simulink model "PV_SEPIC"  (R2025a)
settings: Solver=FixedStepAuto  StartTime=0.0  StopTime=3  RelTol=1e-3
undefined symbols (not defined in the file): Down, sigbuilder_block, Up
libraries: spsSeriesRLCBranchLib x6, spsVoltageMeasurementLib x3, spsGroundLib x2, eePwmGenerator x2, spsCurrentMeasurementLib x1, spsDiodeLib x1, spsMosfetLib x1, slpidlib x1, spsPVArrayLib x1, simulink x1, sps_lib x1
settings Model: Creator=gamezebra  LastModifiedBy=gamezebra

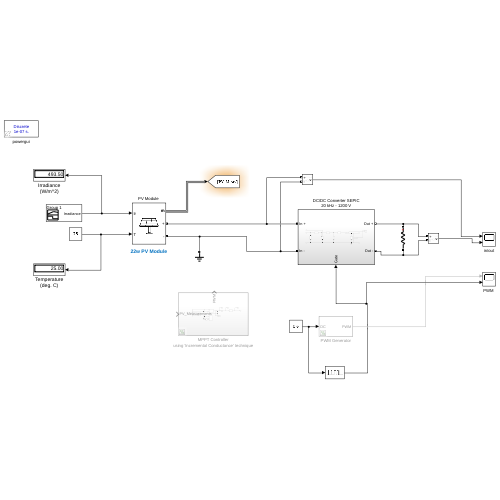
[thumbnail: Simulink's stored preview of the top-level diagram]
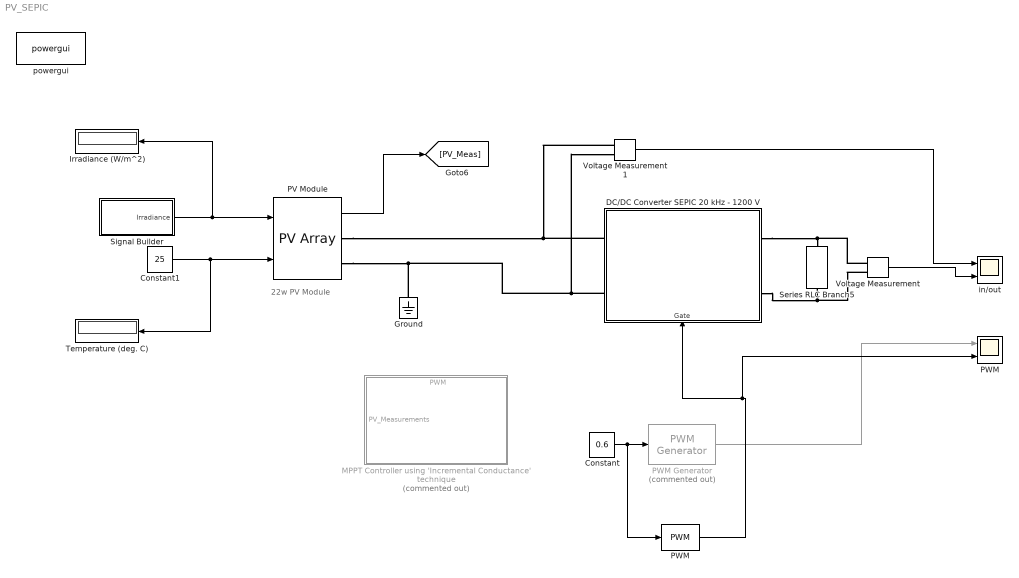
== system PV_SEPIC ==
  note: 22w PV Module
  Constant : Constant  Value=0.6
  Constant1 : Constant  Value=25
  DC/DC Converter SEPIC 20 kHz - 1200 V : Subsystem
      settings: PortSchema="{\"entries\":[{\"content\":{\"sides\":[{\"content\":{\"connectorIds\":[\"LConn1\",\"LConn2\"]},\"type\":\"ConnectorPlacement.EquallySpacedRectSide\",\"uuid\":\"91feb529-5820-4edf-8d0e-1c637fed9421\"},{\"content\":{\"connectorIds\":[\"RConn1\",\"RConn2\"],\"side\":\"RIGHT\"},\"type\":\"ConnectorPlacement.EquallySpacedRectSide\",\"uuid\":\"b4099113-c0ef-4c50-8083-88b14b98cc04\"},{\"content\":{\"side\":\"TOP\"},\"type\":\"ConnectorPlacement.EquallySpacedRectSide\",\"uuid\":\"250c6351-2de3-43d7-b6c9-3c3ed0452184\"},{\"content\":{\"connectorIds\":[\"In1\"],\"side\":\"BOTTOM\"},\"type\":\"ConnectorPlacement.EquallySpacedRectSide\",\"uuid\":\"484af620-bbf2-4328-991e-a08b15b59058\"}]},\"type\":\"ConnectorPlacement.EquallySpacedConnector\",\"uuid\":\"7041a545-1967-46d5-8643-e26f6c990daf\"}],\"packageUris\":[\"http://schema.mathworks.com/mf0/Connector/R2020b\"],\"version\":\"1.0\"}"
  Ground : spsGroundLib/Ground  LConnTagsString=a
  Irradiance (W/m^2) : Display
      settings: Format=bank  Decimation=1000
  MPPT Controller using 'Incremental Conductance' technique : Subsystem  Commented=on
      settings: PortSchema="{\"entries\":[{\"content\":{\"sides\":[{\"content\":{\"connectorIds\":[\"In1\"]},\"type\":\"ConnectorPlacement.EquallySpacedRectSide\",\"uuid\":\"beb56f4d-244a-4861-aa2c-056548243ef9\"},{\"content\":{\"side\":\"RIGHT\"},\"type\":\"ConnectorPlacement.EquallySpacedRectSide\",\"uuid\":\"efb26265-76c3-4ef7-8964-6d49d0ce5848\"},{\"content\":{\"connectorIds\":[\"Out1\"],\"side\":\"TOP\"},\"type\":\"ConnectorPlacement.EquallySpacedRectSide\",\"uuid\":\"f52004c3-ad48-43ff-bda9-03bf57742bdf\"}]},\"type\":\"ConnectorPlacement.EquallySpacedConnector\",\"uuid\":\"0b23e1d0-3529-41b8-bd5c-87ef798e8ebf\"}],\"packageUris\":[\"http://schema.mathworks.com/mf0/Connector/R2020b\"],\"version\":\"1.0\"}"
  "PV Module " : spsPVArrayLib/PV Array  Npar=1  Nser=1  PlotType=one module @ 25 deg.C & specified irradiances  S_vec="[ 1000  500  200 ]"  Temp_C_vec=25  ModuleName=User-defined  PlotWhenSelected=off  Pm=21.6138  Ncell=30  Voc=17.76  Isc=1.5  Vm=16.3  Im=1.326  beta_Voc_pc=-0.37  alpha_Isc_pc=0.07  beta_Voc=-0.065712  alpha_Isc=0.00105  IL=1.5  I0=2.021e-11  nI=1.0007  Rsh=187.3567  Rs=0.40236  RobustModel=off  RobustCellTemperature=313.3991  BAL=on  Tc=1e-6  Tfilter=5e-5
  PWM : simulink/Discontinuities/PWM  DisableCoverage=on  Period=1/100000  InitialDelay=0  DisallowZeroDutyCycle=off  RunAtFixedTimeIntervals=on  SampleTime=0.0000001
  "PWM " : Scope  NumInputPorts=2
      settings: Title=PWM  ActiveDisplayYMinimum=0.19673605992835486  ActiveDisplayYMaximum=1.3583645624515657  YLabel=Amplitudo
  PWM Generator : eePwmGenerator/PWM Generator  Commented=on  CarrCount=Up-Down  Tper=1/20000  Tdelay=0  Ts=0.001
  Series RLC Branch5 : spsSeriesRLCBranchLib/Series RLC Branch  LConnTagsString=__new0  RConnTagsString=__new0  BranchType=R  Resistance=25  Inductance=1e-3  SetiL0=off  InitialCurrent=0  Capacitance=5000e-6  Setx0=off  InitialVoltage=0  Measurements=None
  Signal Builder : Subsystem  Tag=STV Subsys  LoadFcn=sigbuilder_block('load');  StartFcn=sigbuilder_block('start');  StopFcn=sigbuilder_block('stop');  ClipboardFcn=sigbuilder_block('clipboard');  mask(Sigbuilder block){tuvar=[0:10]}
      mask help: Simulink:masks:SigbuilderBlock_MD
      mask init:
      | if ~strcmp(get_param(bdroot(gcbh),'SimulationStatus'),'stopped') tuvar = sigbuilder_block('maskInit'); end
      settings: CopyFcn=sigbuilder_block('copy');  DeleteFcn=sigbuilder_block('delete');  ModelCloseFcn=sigbuilder_block('modelClose');  PreSaveFcn=sigbuilder_block('preSave');  PauseFcn=sigbuilder_block('pause');  ContinueFcn=sigbuilder_block('continue');  NameChangeFcn=sigbuilder_block('namechange');  OpenFcn=sigbuilder_block('open',[316.5 171.75 805.5 485.25 ]);  CloseFcn=sigbuilder_block('close');
      mask Display: plot(0, 0, 100, 100,[2, 2, 32, 32, 2], [68, 8, 8, 68, 68],[32, 2], [38, 38], [32, 19, 2],[53, 60, 44], [32, 17, 17, 2],[16, 16, 31, 31]);txt = getActiveGroup(gcbh);text(2, 100, txt,'verticalAlignment', 'top');
  Temperature (deg. C) : Display
      settings: Format=bank  Decimation=1000
  Voltage Measurement : spsVoltageMeasurementLib/Voltage Measurement  PhasorSimulation=off  OutputType=Complex  PSBequivalent=0
  Voltage Measurement1 : spsVoltageMeasurementLib/Voltage Measurement  PhasorSimulation=off  OutputType=Complex  PSBequivalent=0
  in/out : Scope  NumInputPorts=2
      settings: Title=PWM  ActiveDisplayYMinimum=-2.7461577742739314  ActiveDisplayYMaximum=24.715419991693636  YLabel=Amplitudo  DataLoggingVariableName=ScopeData3
  powergui : sps_lib/powergui  Priority=1  SimulationMode=Discrete  SampleTime=0.0000001  frequency=60  Iterations=50  frequencyindice=0  Pbase=100e6  ErrMax=1e-4  UnitsV=kV  UnitsW=MW  buscounter=0  FunctionMessages=off  echomessages=off  EnableUseOfTLC=off  CurrentSourceSwitches=off  DisableSnubberDevices=off  DisableRonSwitches=off  DisableVfSwitches=off  DisplayEquations=off  AutomaticDiscreteSolvers=off  SolverType=Tustin/Backward Euler (TBE)  Interpol=off  ExternalGateDelay=off  methode=off  Ts=100  x0status=blocks  SPID=on  SwTol=0  HookPort=off  NonlinearTolerance=1e-4  nMaxIteration=100  ContinueOnMaxIteration=off  RestoreLinks=warning  ResistiveCurrentMeasurement=off  Frange=[0:2:500]  Ylog=off  Xlog=on  ShowGrid=off  save=off  variable=ZData  structure=0  ZoomFFT=off  StartTime=0.0  cycles=1  DisplayStyle=1  fundamental=60  FreqAxis=off  MaxFrequency=1000  frequencyindicesteady=1  RmsSteady=1  display=off
  wires:
  PWM Generator/1 -> "PWM "/1
  Constant/1 -> PWM/1, PWM Generator/1
  Voltage Measurement1/1 -> in/out/1
  Voltage Measurement/1 -> in/out/2
  "PV Module "/1 -> [PV_Meas]
  Signal Builder/1(Irradiance) -> "PV Module "/1, Irradiance (W/m^2)/1
  Constant1/1 -> "PV Module "/2, Temperature (deg. C)/1
  PWM/1 -> "PWM "/2, DC/DC Converter SEPIC 20 kHz - 1200 V/1(Gate)
  connections:
  DC/DC Converter SEPIC 20 kHz - 1200 V/LConn1 -- "PV Module "/RConn1 -- Voltage Measurement1/LConn1
  DC/DC Converter SEPIC 20 kHz - 1200 V/RConn1 -- Voltage Measurement/LConn1 -- Series RLC Branch5/LConn1
  DC/DC Converter SEPIC 20 kHz - 1200 V/RConn2 -- Voltage Measurement/LConn2 -- Series RLC Branch5/RConn1
  DC/DC Converter SEPIC 20 kHz - 1200 V/LConn2 -- Ground/LConn1 -- "PV Module "/RConn2 -- Voltage Measurement1/LConn2

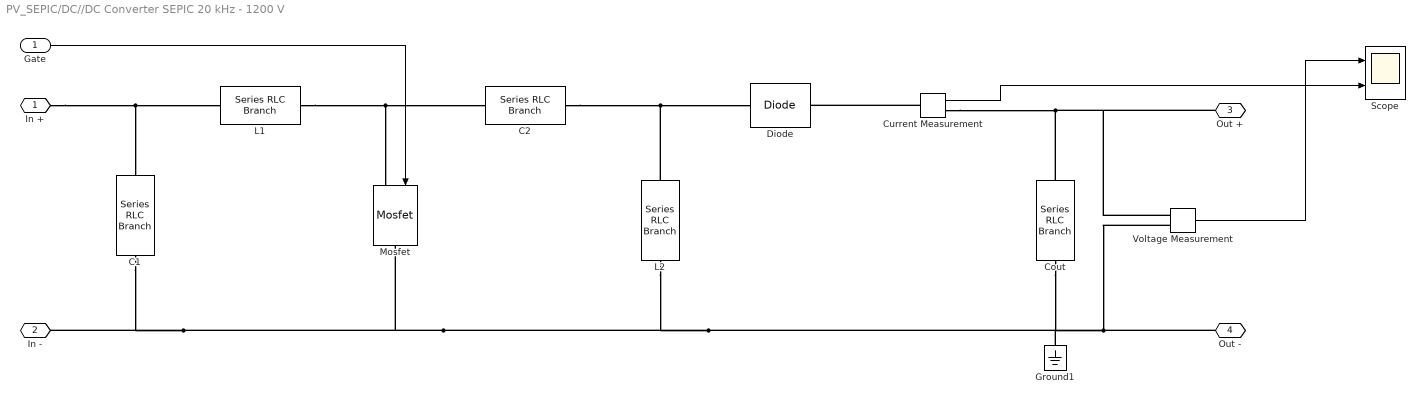
== system PV_SEPIC/DC//DC Converter SEPIC 20 kHz - 1200 V ==
  Gate : Inport
  C1 : spsSeriesRLCBranchLib/Series RLC Branch  LConnTagsString=__new0  RConnTagsString=__new0  BranchType=RC  Resistance=0.01  Inductance=1e-3  SetiL0=off  InitialCurrent=0  Capacitance=0.0001  Setx0=off  InitialVoltage=0  Measurements=None
  C2 : spsSeriesRLCBranchLib/Series RLC Branch  LConnTagsString=__new0  RConnTagsString=__new0  BranchType=C  Resistance=1  Inductance=1e-3  SetiL0=off  InitialCurrent=0  Capacitance=0.00001  Setx0=off  InitialVoltage=0  Measurements=None
  Cout : spsSeriesRLCBranchLib/Series RLC Branch  LConnTagsString=__new0  RConnTagsString=__new0  BranchType=RC  Resistance=0.01  Inductance=16.8e-3  SetiL0=off  InitialCurrent=0  Capacitance=0.0001  Setx0=off  InitialVoltage=0  Measurements=None
  "Current Measurement " : spsCurrentMeasurementLib/Current Measurement  PhasorSimulation=off  OutputType=Complex  PSBequivalent=0
  "Diode " : spsDiodeLib/Diode  Ron=0.001  Lon=0  Vf=0.5  IC=0  UseSnubber=0  Rs=500  Cs=250e-9  Measurements=off
  Ground1 : spsGroundLib/Ground  LConnTagsString=a
  L1 : spsSeriesRLCBranchLib/Series RLC Branch  LConnTagsString=__new0  RConnTagsString=__new0  BranchType=RL  Resistance=0.2  Inductance=0.0002  SetiL0=off  InitialCurrent=0  Capacitance=1e-6  Setx0=off  InitialVoltage=0  Measurements=None
  L2 : spsSeriesRLCBranchLib/Series RLC Branch  LConnTagsString=__new0  RConnTagsString=__new0  BranchType=RL  Resistance=0.2  Inductance=0.0002  SetiL0=off  InitialCurrent=0  Capacitance=1e-6  Setx0=off  InitialVoltage=0  Measurements=None
  Mosfet : spsMosfetLib/Mosfet  Ron=0.1  Lon=0  Rd=0.01  Vfd=0  IC=0  Rs=1e5  Cs=inf  Measurements=off
  Scope : Scope  NumInputPorts=2
      settings: Title=Tegangan Keluaran Konverter SEPIC  ActiveDisplayYMinimum=-151.86738214367281  ActiveDisplayYMaximum=1366.8064463408562  YLabel=Tegangan (Volts)
  "Voltage Measurement " : spsVoltageMeasurementLib/Voltage Measurement  PhasorSimulation=off  OutputType=Complex  PSBequivalent=0
  In + : PMIOPort  Side=Left
  In - : PMIOPort  Port=2  Side=Left
  Out + : PMIOPort  Port=3  Side=Right
  Out - : PMIOPort  Port=4  Side=Right
  wires:
  Gate/1 -> Mosfet/1
  "Current Measurement "/1 -> Scope/2
  "Voltage Measurement "/1 -> Scope/1
  connections:
  Out -/RConn1 -- Cout/RConn1 -- Ground1/LConn1 -- L2/RConn1 -- Mosfet/RConn1 -- C1/RConn1 -- In -/RConn1 -- "Voltage Measurement "/LConn2
  L1/RConn1 -- C2/LConn1 -- Mosfet/LConn1
  C2/RConn1 -- L2/LConn1 -- "Diode "/LConn1
  Cout/LConn1 -- "Voltage Measurement "/LConn1 -- Out +/RConn1 -- "Current Measurement "/RConn1
  In +/RConn1 -- L1/LConn1 -- C1/LConn1
  "Current Measurement "/LConn1 -- "Diode "/RConn1

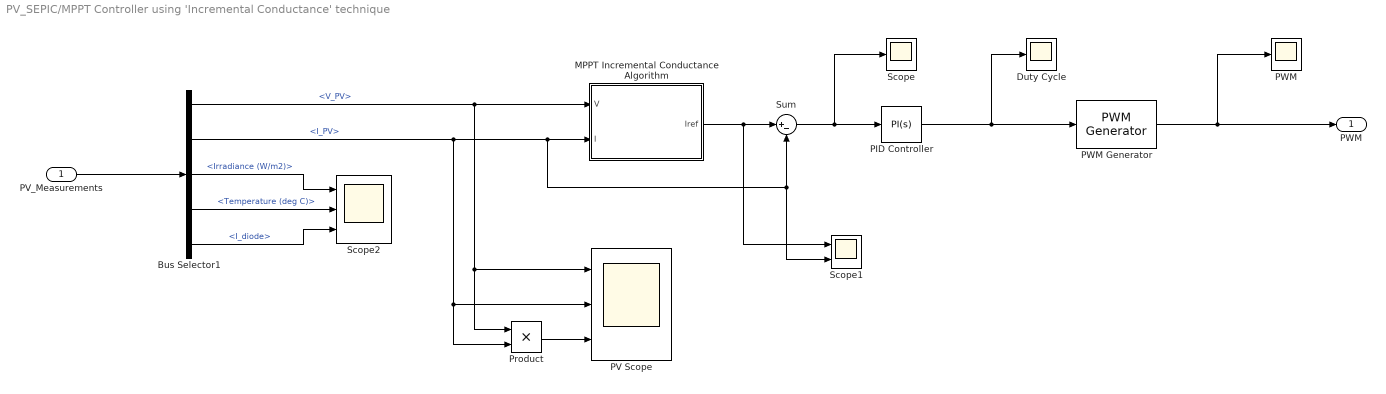
== system PV_SEPIC/MPPT Controller using 'Incremental Conductance' technique ==
  PV_Measurements : Inport
  Bus Selector1 : BusSelector  OutputSignals=V_PV,I_PV,Irradiance (W/m2),Temperature (deg C),I_diode
  Duty Cycle : Scope
      settings: Title=Duty Cycle dari MPPT  ActiveDisplayYMinimum=-0.125  ActiveDisplayYMaximum=1.125  YLabel=Amplitudo  DataLoggingVariableName=ScopeData2
  MPPT Incremental Conductance Algorithm : MATLAB Function  TreatAsAtomicUnit=on
  PID Controller : slpidlib/PID Controller  Controller=PI  Form=Parallel  TimeDomain=Continuous-time  UseExternalTs=off  SampleTime=-1  IntegratorMethod=Forward Euler  FilterMethod=Forward Euler  ControllerParametersSource=internal  P=0.05  I=0.05*(1/1000000)  UseKiTs=off  D=0  UseExternalDerivativeSource=off  N=100  UseFilter=on  TunerSelectOption=Transfer Function Based (PID Tuner App)  InitialConditionSource=internal  InitialConditionForIntegrator=0  InitialConditionForFilter=0  DifferentiatorICPrevScaledInput=0  ExternalReset=none  TrackingMode=off  Kt=1  LimitOutput=on  SatLimitsSource=internal  UpperSaturationLimit=1  LowerSaturationLimit=0  LinearizeAsGain=on  AntiWindupMode=none  Kb=1  LimitIntegrator=off  UpperIntegratorSaturationLimit=inf  LowerIntegratorSaturationLimit=-inf  POutMin=[]  POutMax=[]  IOutMin=[]  IOutMax=[]  DOutMin=[]  DOutMax=[]  NOutMin=[]  NOutMax=[]  SumOutMin=[]  SumOutMax=[]  SaturationOutMin=[]  SaturationOutMax=[]  PParamMin=[]  PParamMax=[]  IParamMin=[]  IParamMax=[]  DParamMin=[]  DParamMax=[]  NParamMin=[]  NParamMax=[]  KbParamMin=[]  KbParamMax=[]  KtParamMin=[]  KtParamMax=[]  KbOutMin=[]  KbOutMax=[]  KtOutMin=[]  KtOutMax=[]  IntegratorOutMin=[]  IntegratorOutMax=[]  FilterOutMin=[]  FilterOutMax=[]  SumI1OutMin=[]  SumI1OutMax=[]  SumI2OutMin=[]  SumI2OutMax=[]  SumI3OutMin=[]  SumI3OutMax=[]  SumI4OutMin=[]  SumI4OutMax=[]  SumDOutMin=[]  SumDOutMax=[]  DifferentiatorOutMin=[]  DifferentiatorOutMax=[]  FilterDiffOutCoefMin=[]  FilterDiffOutCoefMax=[]  ReciprocalOutMin=[]  ReciprocalOutMax=[]  SumDenOutMin=[]  SumDenOutMax=[]  SumNumOutMin=[]  SumNumOutMax=[]  DivideOutMin=[]  DivideOutMax=[]  UdiffTsProdOutMin=[]  UdiffTsProdOutMax=[]  NTsProdOutMin=[]  NTsProdOutMax=[]  UintegralTsProdOutMin=[]  UintegralTsProdOutMax=[]  UngainTsProdOutMin=[]  UngainTsProdOutMax=[]  ClampingZeroOutDataTypeStr=Inherit: Inherit via back propagation  ClampingZeroOutMin=[]  ClampingZeroOutMax=[]  FilterDenConstantOutDataTypeStr=Inherit: Inherit via back propagation  FilterDenConstantOutMin=[]  FilterDenConstantOutMax=[]  PCopyOutDataTypeStr=Inherit: Inherit via back propagation  PCopyOutMin=[]  PCopyOutMax=[]  NCopyOutDataTypeStr=Inherit: Inherit via back propagation  NCopyOutMin=[]  NCopyOutMax=[]  IntegratorContinuousStateAttributes=''  IntegratorStateMustResolveToSignalObject=off  IntegratorRTWStateStorageClass=Auto  FilterContinuousStateAttributes=''  FilterStateMustResolveToSignalObject=off  FilterRTWStateStorageClass=Auto  ParallelPVariant=InternalParameters  IdealPVariant=Disabled  IVariant=InternalParameters  DVariant=Disabled  IntegratorVariant=Continuous  SatVariant=Enabled  AWVariant=Passthrough  PCopyVariant=Disabled  TRVariant=Disabled  FdbkBlocksVariant=Forward  IdealPFdbkVariant=Disabled  SatFdbkVariant=Disabled  DerivativeFilterVariant=Disabled  NVariant=Disabled  NCopyVariant=Disabled_SignalSpec  FilterICVariant=Disabled  IntegratorICVariant=InternalICs  ExternalResetVariant=Disabled  TRSumVariant=Passthrough  SumFdbkVariant=Disabled  SumVariant=Sum_PI  TsampFilterVariant=InternalTs  TsampNgainVariant=Passthrough  TsampIntegralVariant=Disabled_SignalSpec  ExternalSaturationOutDataTypeStr=Inherit: Same as second input  DerivativeSourceVariant=Disabled  PreIntVariant=InternalPreInt
  PV Scope : Scope  NumInputPorts=3
      settings: Title=Tegangan PV  ActiveDisplayYMinimum=-112.5443  ActiveDisplayYMaximum=1023.37415  YLabel=Tegangan (Volts)
  "PWM " : Scope
      settings: Title=PWM  ActiveDisplayYMinimum=-0.12499999999999997  ActiveDisplayYMaximum=1.125  YLabel=Amplitudo
  PWM Generator : eePwmGenerator/PWM Generator  CarrCount=Up-Down  Tper=1/20000  Tdelay=0  Ts=1e-6
  Product : Product
  Scope : Scope
      settings: Title=Selisih Nilai Arus antara Arus Maksimum PV (Iref) dan Arus PV Aktual (Ipv)  ActiveDisplayYMinimum=-41.63782  ActiveDisplayYMaximum=28.53567  YLabel=Arus (Ampere)  DataLoggingVariableName=ScopeData2
  Scope1 : Scope  NumInputPorts=2
      settings: Title=Arus MPPT (Iref) dan Arus PV Aktual (Ipv)  ActiveDisplayYMinimum=-13.35212  ActiveDisplayYMaximum=79.26135  YLabel=Current (Amperes)
  Scope2 : Scope  NumInputPorts=3
      settings: Title=Irradiance  ActiveDisplayYMinimum=437.5  ActiveDisplayYMaximum=1062.5  YLabel=(W/m^2)
  Sum : Sum  Inputs=|+-
  PWM : Outport
  wires:
  PWM Generator/1 -> "PWM "/1, PWM/1
  Product/1 -> PV Scope/3
  Bus Selector1/1 -> MPPT Incremental Conductance Algorithm/1(V), PV Scope/1, Product/1  "<V_PV>"
  Bus Selector1/2 -> PV Scope/2, Product/2, MPPT Incremental Conductance Algorithm/2(I), Scope1/2, Sum/2  "<I_PV>"
  Bus Selector1/3 -> Scope2/1  "<Irradiance (W/m2)>"
  Bus Selector1/5 -> Scope2/3  "<I_diode>"
  Bus Selector1/4 -> Scope2/2  "<Temperature (deg C)>"
  PV_Measurements/1 -> Bus Selector1/1
  PID Controller/1 -> Duty Cycle/1, PWM Generator/1
  MPPT Incremental Conductance Algorithm/1(Iref) -> Scope1/1, Sum/1
  Sum/1 -> Scope/1, PID Controller/1

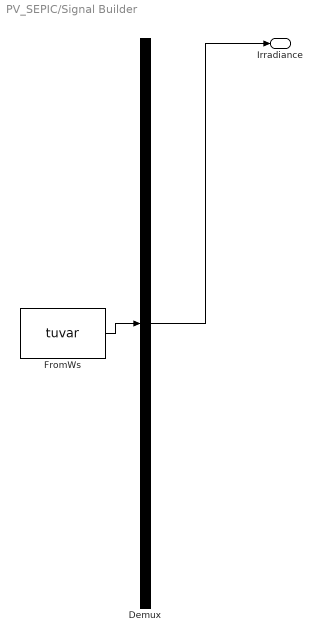
== system PV_SEPIC/Signal Builder ==
  Demux : Demux  Tag=STV Demux  Outputs=1
      settings: DisplayOption=none
  FromWs : FromWorkspace  Tag=STV FromWs  VariableName=tuvar
      SigBuilderData=|
      | common.afterFinalStr = 'Extrapolate'
      | common.sampleTime = 0
      | dataSet.timeRange = [0 2]
      | dataSet.name = 'Group 1'
      | sbobj.Groups.Name = 'Group 1'
      | sbobj.Groups.Signals.Name = 'Irradiance'
      | sbobj.Groups.Signals.XData = [0 0.48 0.52 0.98 0.98 1.235 1.48 1.66 1.66 2]
      | sbobj.Groups.Signals.YData = [493.5 493.5 802 802 801 538 626 927 928 926]
      | sbobj.Groups.TimeRange = [0 2]
  Irradiance : Outport  Tag=STV Outport
  wires:
  Demux/1 -> Irradiance/1
  FromWs/1 -> Demux/1

== matlab function PV_SEPIC/MPPT Controller using 'Incremental Conductance' technique/MPPT Incremental Conductance Algorithm ==
  settings: updateMethod=DISCRETE
  data: V input; Iref output; I input
function Iref = MPPT_INC(V,I)

Irefinit = 0;
Irefmax = 70;
Irefmin = 0;
deltaIref = 0.0008;

persistent Vold Iold Irefold

if isempty(Vold)
    Vold = 0;
    Iold = 0;
    Irefold = Irefinit;
end

dV = V - Vold;
dI = I - Iold;

if dV == 0
    if dI == 0
        Iref = Irefold;
    elseif dI > 0
        Iref = Irefold + (deltaIref);
    else
        Iref = Irefold - (deltaIref);
    end
    else
    if dI/dV == -I/V
        Iref = Irefold;
    elseif dI/dV > -I/V
        Iref = Irefold - (deltaIref);
    else
        Iref = Irefold + (deltaIref);
    end
end

if Iref >= Irefmax || Iref <= Irefmin
    Iref = Irefold;
end

Irefold = Iref;
Vold = V;
Iold = I;
